simulink model "PubIfDecisionLSM_MDL"  (R2020b)
settings: configuration reference "DspaceConfig" (kept outside this file)
PostLoadFcn:
  | if any(exist('dsrtsu_mdlpostloadfcn', 'file') ~= 0), dsrtsu_mdlpostloadfcn('Execute', bdroot); end
InitFcn:
  | , if any(exist('rtifpga_mdlclblib', 'file') ~= 0), rtifpga_mdlclblib('Init', bdroot); end,
  | , if any(exist('dsmpb_private', 'file') ~= 0), dsmpb_private('dsmpb_mdlclblib', 'Init', bdroot); end,
values from neighbouring files (symbols this model uses):
  P_LSM_ALC_Enable = 0.0    [LSM_Parameter.sldd]
  P_LSM_AwayEdge_offset = 0.1    [LSM_Parameter.sldd]
  P_LSM_CentValidErr = 1.0    [LSM_Parameter.sldd]
  P_LSM_DOP_C0_EN_Limit = 0.8    [LSM_Parameter.sldd]
  P_LSM_DOP_C0_out_Limit = 2.0    [LSM_Parameter.sldd]
  P_LSM_DOP_C1_EN_Limit : value not decoded    [LSM_Parameter.sldd]
  P_LSM_DOP_C1_out_Limit : value not decoded    [LSM_Parameter.sldd]
  P_LSM_DOP_C1AndC2_Lim_X : value not decoded    [LSM_Parameter.sldd]
  P_LSM_DOP_C2_EN_Limit : value not decoded    [LSM_Parameter.sldd]
  P_LSM_DOP_C2_out_Limit : value not decoded    [LSM_Parameter.sldd]
  P_LSM_DOP_In_Pre2Dop_Dis = 1.0    [LSM_Parameter.sldd]
  P_LSM_DOP_Out_Pre2Dop_Dis = 2.0    [LSM_Parameter.sldd]
  P_LSM_DOP_PreDis_X : value not decoded    [LSM_Parameter.sldd]
  P_LSM_DOP_PreDis_Y : value not decoded    [LSM_Parameter.sldd]
  P_LSM_DOPEnableSW = 1.0    [LSM_Parameter.sldd]
  P_LSM_DOPValid_CheckTime = 0.06    [LSM_Parameter.sldd]
  P_LSM_DoubleLine_Curr2Cent_Dislimit = 0.5    [LSM_Parameter.sldd]
  P_LSM_DoubleLine_Dop2Cent_Dislimit = 0.5    [LSM_Parameter.sldd]
  P_LSM_DoubleLine_DOPOut_C1 : value not decoded    [LSM_Parameter.sldd]
  P_LSM_DoubleLine_Pre2Cent_Dislimit = 1.0    [LSM_Parameter.sldd]
  P_LSM_Error_Limit = 0.5    [LSM_Parameter.sldd]
  P_LSM_IFV2CenterAxis = 0.0    [LSM_Parameter.sldd]
  P_LSM_IFV2RearAxis = 0.0    [LSM_Parameter.sldd]
  P_LSM_Line2Edge_limit = 0.5    [LSM_Parameter.sldd]
  P_LSM_Line_Error = 0.1    [LSM_Parameter.sldd]
  P_LSM_LineSTD_Limit = 0.15    [LSM_Parameter.sldd]
  P_LSM_NOH_Switch = 0.0    [LSM_Parameter.sldd]
  P_LSM_OTL_C0_Factor = 1.0    [LSM_Parameter.sldd]
  P_LSM_OTL_C1_Factor = 0.5    [LSM_Parameter.sldd]
  P_LSM_OTL_C2_Factor = 0.5    [LSM_Parameter.sldd]
  P_LSM_Pre2OnlyLineDis = 5.0    [LSM_Parameter.sldd]
  P_LSM_Pre_t = 0.0    [LSM_Parameter.sldd]
  P_LSM_SingleLine_Cent2Edge_Dislimit = 100.0    [LSM_Parameter.sldd]
  P_LSM_SingleLine_Curr2Cent_Dislimit = 0.2    [LSM_Parameter.sldd]
  P_LSM_SingleLine_Dop2Cent_Dislimit = 0.2    [LSM_Parameter.sldd]
  P_LSM_SingleLine_DOPOut_C1 : value not decoded    [LSM_Parameter.sldd]
  P_LSM_SingleLine_Pre2Cent_Dislimit = 0.5    [LSM_Parameter.sldd]
  P_LSM_TJALimitSpd = 60.0    [LSM_Parameter.sldd]
undefined symbols (not defined in the file or in its folder): P_lCS_IFV2CenterAxis, P_LCS_IFV2RearAxis, P_LSM_EntryEdge_offset, P_LSM_EntryLnChngEnSwitch, P_LSM_EntryVanishDis, P_LSM_LinetLostTime, P_LSM_LineWijCal_C12, P_LSM_LineWijCal_C13, P_LSM_MapValid_ErrorSwitch, P_LSM_PosLineLcFac, P_LSM_SpdLim_Stub_Spd, P_LSM_SpdLim_StubLength, P_LSM_SpdTurnAlarm
libraries: simulink x324, TrueDurationTime x11
(part 8 of 25)

== system PubIfDecisionLSM_MDL/Subsystem1/TargetLineCalc_20ms/TargetLineCalc/DetectChange ==
  OTLCount : Inport
  Relational Operator : RelationalOperator  Operator=~=  OutDataTypeStr=boolean  RndMeth=Simplest
  Unit Delay49 : UnitDelay  InitialCondition=uint8(0)  SampleTime=-1  HasFrameUpgradeWarning=on
  Out1 : Outport
  wires:
  Unit Delay49/1 -> Relational Operator/1
  OTLCount/1 -> Relational Operator/2, Unit Delay49/1
  Relational Operator/1 -> Out1/1

== system PubIfDecisionLSM_MDL/Subsystem1/TargetLineCalc_20ms/TargetLineCalc/DetectIncrease ==
  LeftOffset_b : Inport
  Relational Operator : RelationalOperator  Operator=>  OutDataTypeStr=boolean  RndMeth=Simplest
  Unit Delay67 : UnitDelay  SampleTime=-1  HasFrameUpgradeWarning=on
  Out : Outport
  wires:
  Unit Delay67/1 -> Relational Operator/2
  LeftOffset_b/1 -> Unit Delay67/1, Relational Operator/1
  Relational Operator/1 -> Out/1

== system PubIfDecisionLSM_MDL/Subsystem1/TargetLineCalc_20ms/TargetLineCalc/DetectIncrease1 ==
  RightOffset_b : Inport
  Relational Operator : RelationalOperator  Operator=>  OutDataTypeStr=boolean  RndMeth=Simplest
  Unit Delay67 : UnitDelay  SampleTime=-1  HasFrameUpgradeWarning=on
  Out : Outport
  wires:
  Unit Delay67/1 -> Relational Operator/2
  RightOffset_b/1 -> Unit Delay67/1, Relational Operator/1
  Relational Operator/1 -> Out/1

== system PubIfDecisionLSM_MDL/Subsystem1/TargetLineCalc_20ms/TargetLineCalc/Subsystem2 ==
  LCKSts : Inport
  Line_State : Inport  Port=2
  vRef : Inport  Port=3
  DOP_Valid : Inport  Port=4
  DOP_C3 : Inport  Port=5
  DOP_C2 : Inport  Port=6
  DOP_C1 : Inport  Port=7
  DOP_C0 : Inport  Port=8
  DOP_Range : Inport  Port=9
  CentLine : Inport  Port=10
  EdgeLine : Inport  Port=11
  kap : Inport  Port=12
  Bus Selector1 : BusSelector  OutputSignals=EdgeConf,EdgeA3,EdgeA2,EdgeA1,EdgeA0
  Bus Selector6 : BusSelector  OutputSignals=PathValid,PathA3,PathA2,PathA1,PathA0,PathRange
  Constant11 : Constant  Value=1.3  OutDataTypeStr=single
  Constant13 : Constant  Value=P_LSM_DoubleLine_Dop2Cent_Dislimit
  Constant14 : Constant  Value=P_LSM_DOP_In_Pre2Dop_Dis
  Constant16 : Constant  Value=P_LSM_SingleLine_Cent2Edge_Dislimit
  Constant17 : Constant  Value=P_LSM_SingleLine_Pre2Cent_Dislimit
  Constant18 : Constant  Value=P_LSM_SingleLine_Curr2Cent_Dislimit
  Constant19 : Constant  Value=P_LSM_DoubleLine_Pre2Cent_Dislimit
  Constant20 : Constant  Value=P_LSM_DoubleLine_Curr2Cent_Dislimit
  Constant21 : Constant  Value=P_LSM_SingleLine_Dop2Cent_Dislimit
  Constant22 : Constant  Value=P_LSM_DOP_Out_Pre2Dop_Dis
  Constant23 : Constant  Value=P_LSM_DOPValid_CheckTime
  Constant3 : Constant  Value=P_LSM_DOP_C0_EN_Limit
  Constant6 : Constant  Value=P_LSM_DOP_C0_out_Limit
  Constant9 : Constant  Value=1.3  OutDataTypeStr=single
  Gain1 : Gain  Gain=3.6
  Gain2 : Gain  Gain=1.03
  Gain3 : Gain  Gain=3.6
  Gain4 : Gain  Gain=1.03
  LineSelect1 : MATLAB Function  TreatAsAtomicUnit=on
  MATLAB Function : MATLAB Function  TreatAsAtomicUnit=on
  Relational Operator3 : RelationalOperator  Operator=>  OutDataTypeStr=boolean  RndMeth=Simplest
  Selector{1..5,13} (6 alike) : Selector  InputPortWidth=3  IndexOptions=Index vector (dialog)  Indices=2  OutputSizes=1
  Sum : Sum  Inputs=|++
  Sum1 : Sum  Inputs=|++
  TJA_Line_Select : Stateflow chart  TreatAsAtomicUnit=on
      settings: PortSchema="{\"entries\":[{\"content\":{\"sides\":[{\"content\":{\"connectorIds\":[\"In4\",\"In5\",\"In1\",\"In3\",\"In6\",\"In2\"]},\"type\":\"ConnectorPlacement.EquallySpacedRectSide\",\"uuid\":\"94136a59-7eb8-456e-b1b6-1f0641166e38\"},{\"content\":{\"connectorIds\":[\"Out1\",\"Out2\"],\"side\":\"RIGHT\"},\"type\":\"ConnectorPlacement.EquallySpacedRectSide\",\"uuid\":\"664f3682-a903-47ba-a547-cb8bac6665aa\"},{\"content\":{\"connectorIds\":[],\"side\":\"TOP\"},\"type\":\"ConnectorPlacement.EquallySpacedRectSide\",\"uuid\":\"464c275d-d572-4c7f-987d-e7fbd4ad7b48\"},{\"content\":{\"connectorIds\":[],\"side\":\"HIDDEN\"},\"type\":\"ConnectorPlacement.EquallySpacedRectSide\",\"uuid\":\"4c0a197a-3630-40df-8db9-9313a36d3a51\"}]},\"type\":\"ConnectorPlacement.EquallySpacedConnector\",\"uuid\":\"5cfbbf76-c0d2-41e2-9bfb-a7f0229f0d71\"}],\"packageUris\":[\"http://schema.mathworks.com/mf0/Connector/R2020b\"],\"version\":\"1.0\"}"
  TrueDurationTime8 : TrueDurationTime/TrueDurationTime  TCycle=0.02
  Unit Delay : UnitDelay  SampleTime=-1  HasFrameUpgradeWarning=on
  Unit Delay1 : UnitDelay  SampleTime=-1  HasFrameUpgradeWarning=on
  Unit Delay2 : UnitDelay  SampleTime=-1  HasFrameUpgradeWarning=on
  preDisMinTable : Lookup_n-D  NumberOfTableDimensions=1  BreakpointsForDimension1=P_LSM_DOP_PreDis_X  Table=P_LSM_DOP_PreDis_Y  ExtrapMethod=Clip  InternalRulePriority=Speed  RndMeth=Simplest  InputSameDT=on
  preDisMinTable1 : Lookup_n-D  NumberOfTableDimensions=1  BreakpointsForDimension1=P_LSM_DOP_C1AndC2_Lim_X  Table=P_LSM_DOP_C1_EN_Limit  ExtrapMethod=Clip  InternalRulePriority=Speed  RndMeth=Simplest  InputSameDT=on
  preDisMinTable2 : Lookup_n-D  NumberOfTableDimensions=1  BreakpointsForDimension1=P_LSM_DOP_C1AndC2_Lim_X  Table=P_LSM_DOP_C2_EN_Limit  ExtrapMethod=Clip  InternalRulePriority=Speed  RndMeth=Simplest  InputSameDT=on
  preDisMinTable3 : Lookup_n-D  NumberOfTableDimensions=1  BreakpointsForDimension1=P_LSM_DOP_C1AndC2_Lim_X  Table=P_LSM_DOP_C1_out_Limit  ExtrapMethod=Clip  InternalRulePriority=Speed  RndMeth=Simplest  InputSameDT=on
  preDisMinTable4 : Lookup_n-D  NumberOfTableDimensions=1  BreakpointsForDimension1=P_LSM_DOP_C1AndC2_Lim_X  Table=P_LSM_DOP_C2_out_Limit  ExtrapMethod=Clip  InternalRulePriority=Speed  RndMeth=Simplest  InputSameDT=on
  preDisMinTable5 : Lookup_n-D  NumberOfTableDimensions=1  BreakpointsForDimension1=P_LSM_DOP_C1AndC2_Lim_X  Table=P_LSM_DoubleLine_DOPOut_C1  ExtrapMethod=Clip  InternalRulePriority=Speed  RndMeth=Simplest  InputSameDT=on
  preDisMinTable7 : Lookup_n-D  NumberOfTableDimensions=1  BreakpointsForDimension1=P_LSM_DOP_C1AndC2_Lim_X  Table=P_LSM_SingleLine_DOPOut_C1  ExtrapMethod=Clip  InternalRulePriority=Speed  RndMeth=Simplest  InputSameDT=on
  vRef2 : InportShadow  Port=3
  OTL_Valid : Outport
  OTL_C3 : Outport  Port=2
  OTL_C2 : Outport  Port=3
  OTL_C1 : Outport  Port=4
  OTL_C0 : Outport  Port=5
  OTL_Range : Outport  Port=6
  TJA_Line_State : Outport  Port=7
  Line_source : Outport  Port=8
  wires:
  [SpeedKph] -> preDisMinTable7/1, preDisMinTable5/1
  preDisMinTable7/1 -> LineSelect1/27(SingleLine_DOPOut_C1)
  preDisMinTable5/1 -> LineSelect1/28(DoubleLine_DOPOut_C1)
  preDisMinTable2/1 -> MATLAB Function/7(DOP_C2_EN_Limit)
  preDisMinTable1/1 -> MATLAB Function/6(DOP_C1_EN_Limit)
  preDisMinTable3/1 -> MATLAB Function/9(DOP_C1_out_Limit)
  [SpeedKph] -> preDisMinTable1/1, preDisMinTable2/1, preDisMinTable3/1, preDisMinTable4/1
  Unit Delay2/1 -> MATLAB Function/14(dy_pre)
  LineSelect1/7(dy_pre) -> Unit Delay2/1
  Unit Delay1/1 -> MATLAB Function/15(Y_DOP)
  LineSelect1/5(Cent2DOP_flag) -> TJA_Line_Select/6(Cent2DOP_flag)
  LineSelect1/6(DOP2Cent_flag) -> TJA_Line_Select/2(DOP2Cent_flag)
  Unit Delay/1 -> MATLAB Function/1(TJA_Line)
  MATLAB Function/2(DOP_Out_Enable) -> LineSelect1/31(DOP_OUT)  "LSM_DOP_Out"
  Constant23/1 -> Relational Operator3/2
  Constant22/1 -> MATLAB Function/12(DOP_Out_Pre2Dop_Dis)
  Constant21/1 -> LineSelect1/26(SingleLine_Dop2Cent_Dislimit)
  Constant18/1 -> LineSelect1/25(SingleLine_Curr2Cent_Dislimit)
  Constant17/1 -> LineSelect1/24(SingleLine_Pre2Cent_Dislimit)
  Constant16/1 -> LineSelect1/23(SingleLine_Cent2Edge_Dislimit)
  LineSelect1/4(DOP2Off_flag) -> TJA_Line_Select/3(DOP2Off_flag)
  LineSelect1/3(Cent2Off_flag) -> TJA_Line_Select/1(Cent2Off_flag)
  LineSelect1/2(Off2DOP_flag) -> TJA_Line_Select/5(Off2DOP_flag)
  LineSelect1/1(Off2Cent_flag) -> TJA_Line_Select/4(Off2Cent_flag)
  kap/1 -> LineSelect1/3(kap)
  Constant13/1 -> LineSelect1/22(DoubleLine_Dop2Cent_Dislimit)
  Constant20/1 -> LineSelect1/21(DoubleLine_Curr2Cent_Dislimit)
  Constant19/1 -> LineSelect1/20(DoubleLine_Pre2Cent_Dislimit)
  EdgeLine/1 -> Bus Selector1/1
  Bus Selector1/1 -> LineSelect1/15(VisEdgeConf)  "<EdgeConf>"
  Bus Selector1/3 -> LineSelect1/17(VisEdgeA2)  "<EdgeA2>"
  Bus Selector1/5 -> LineSelect1/19(VisEdgeA0)  "<EdgeA0>"
  Bus Selector1/2 -> LineSelect1/16(VisEdgeA3)  "<EdgeA3>"
  Bus Selector1/4 -> LineSelect1/18(VisEdgeA1)  "<EdgeA1>"
  [DOP_C2] -> LineSelect1/12(bOTL)
  [DOP_C1] -> LineSelect1/13(cOTL)
  [DOP_C0] -> LineSelect1/14(dOTL)
  [DOP_C3] -> LineSelect1/11(aOTL)
  Bus Selector6/3 -> Selector2/1  "<PathA2>"
  Bus Selector6/6 -> Selector5/1  "<PathRange>"
  Bus Selector6/5 -> Selector4/1  "<PathA0>"
  Bus Selector6/1 -> Selector13/1  "<PathValid>"
  Bus Selector6/2 -> Selector1/1  "<PathA3>"
  Bus Selector6/4 -> Selector3/1  "<PathA1>"
  CentLine/1 -> Bus Selector6/1
  Constant14/1 -> MATLAB Function/11(DOP_In_Pre2Dop_Dis)
  LineSelect1/8(Y_DOP) -> Unit Delay1/1
  Line_State/1 -> LineSelect1/2(Line_State)
  Gain1/1 -> Gain2/1
  Sum1/1 -> preDisMinTable/1
  vRef2/1 -> Gain1/1
  Gain2/1 -> Sum1/1
  Constant11/1 -> Sum1/2
  LCKSts/1 -> LineSelect1/4(LCKSts)
  preDisMinTable/1 -> LineSelect1/1(Pre_dis)
  Constant9/1 -> Sum/2
  vRef/1 -> Gain3/1
  Gain4/1 -> Sum/1
  Gain3/1 -> Gain4/1
  Sum/1 -> LineSelect1/29(Vehicle_Speed), [SpeedKph]
  Relational Operator3/1 -> MATLAB Function/13(DOP_Valid)
  TrueDurationTime8/1 -> Relational Operator3/1
  [DOP_Valid] -> TrueDurationTime8/1
  preDisMinTable4/1 -> MATLAB Function/10(DOP_C2_out_Limit)
  Constant6/1 -> MATLAB Function/8(DOP_CO_out_Limit)
  Constant3/1 -> MATLAB Function/5(DOP_CO_EN_Limit)
  TJA_Line_Select/1(TJA_Line) -> TJA_Line_State/1, Unit Delay/1
  MATLAB Function/1(DOP_In_Enable) -> LineSelect1/30(DOP_EN)  "LSM_DOP_EN"
  DOP_C0/1 -> OTL_C0/1, [DOP_C0]
  DOP_Valid/1 -> [DOP_Valid], OTL_Valid/1
  DOP_Range/1 -> OTL_Range/1, [DOP_Range]
  DOP_C1/1 -> OTL_C1/1, [DOP_C1]
  DOP_C2/1 -> OTL_C2/1, [DOP_C2]
  DOP_C3/1 -> OTL_C3/1, [DOP_C3]
  [DOP_C0] -> MATLAB Function/2(DOP_CO)
  [DOP_C1] -> MATLAB Function/3(DOP_C1)
  [DOP_C2] -> MATLAB Function/4(DOP_C2)
  Selector13/1 -> LineSelect1/5(CentLaneValid)
  Selector1/1 -> LineSelect1/6(CentLineA3)
  Selector2/1 -> LineSelect1/7(CentLineA2)
  Selector3/1 -> LineSelect1/8(CentLineA1)
  Selector4/1 -> LineSelect1/9(CentLineA0)
  Selector5/1 -> LineSelect1/10(CentRange)
  TJA_Line_Select/2(TJA_Source) -> Line_source/1

== system PubIfDecisionLSM_MDL/Subsystem1/TargetLineCalc_20ms/TargetLineCalc/Subsystem3 ==
  Intersec_available : Inport
  f_distance : Inport  Port=2  OutDataTypeStr=single
  en_direction : Inport  Port=3  OutDataTypeStr=uint8
  i_rec_lanes_num : Inport  Port=4  OutDataTypeStr=uint8
  i_rec_lanes : Inport  Port=5  OutDataTypeStr=uint8
  nLaneNum : Inport  Port=6  OutDataTypeStr=uint8
  nLaneID : Inport  Port=7  OutDataTypeStr=uint8
  i_mapvalid : Inport  Port=8  OutDataTypeStr=uint8
  i_on_nav_path : Inport  Port=9  OutDataTypeStr=uint8
  " b_vanish_valid" : Inport  Port=10  OutDataTypeStr=boolean
  " Exit_dDisStart" : Inport  Port=11  OutDataTypeStr=single
  ExitLineExist : Inport  Port=12  OutDataTypeStr=uint8
  " Exit_dC0V" : Inport  Port=13  OutDataTypeStr=single
  RoadType : Inport  Port=14  OutDataTypeStr=uint8
  VehInLeftmostLane : Inport  Port=15  OutDataTypeStr=boolean
  VehInRightmostLane : Inport  Port=16  OutDataTypeStr=boolean
  Entry_bIsLineExist : Inport  Port=17
  Entry_dDisStart : Inport  Port=18
  Entry_dC0V : Inport  Port=19
  " f_vanish_pt_dis " : Inport  Port=20
  Subsystem : Subsystem
  Subsystem2 : Subsystem
  Subsystem3 : Subsystem
  PilotRoadSts : Outport  OutDataTypeStr=uint8
  PilotTurnSwSts : Outport  Port=2  OutDataTypeStr=uint8
  PilotSts : Outport  Port=3  OutDataTypeStr=uint8
  LaneChange : Outport  Port=4  OutDataTypeStr=uint8
  LSM_PilotSPL : Outport  Port=5  OutDataTypeStr=uint8
  PilotSPLDist : Outport  Port=6  OutDataTypeStr=uint16
  wires:
  " b_vanish_valid"/1 -> Subsystem2/11(" b_vanish_valid")
  nLaneNum/1 -> Subsystem2/9(nLaneNum)
  VehInLeftmostLane/1 -> Subsystem2/8(VehInLeftmostLane)
  VehInRightmostLane/1 -> Subsystem2/7(VehInRightmostLane)
  RoadType/1 -> Subsystem/3(RoadType)
  nLaneID/1 -> Subsystem2/5(nLaneID), [nLaneID]
  i_on_nav_path/1 -> Subsystem/2(i_on_nav_path)
  " Exit_dC0V"/1 -> Subsystem2/13(Exit_dC0V)
  " Exit_dDisStart"/1 -> Subsystem2/12(" Exit_dDisStart")
  f_distance/1 -> Subsystem2/2(f_distance), Subsystem/5(f_distance)
  Subsystem2/9(rExitStub3) -> Subsystem/14(rExitStub3)
  i_rec_lanes_num/1 -> Subsystem2/10(i_rec_lanes_num)
  i_mapvalid/1 -> Subsystem/1(i_mapvalid)
  i_rec_lanes/1 -> Subsystem2/4(i_rec_lanes)
  ExitLineExist/1 -> Subsystem2/1(Exit_bIsLineExist), Subsystem/4(bIsLineExist)
  en_direction/1 -> Subsystem2/6(en_direction)
  Subsystem2/16(lExitStub3) -> Subsystem/21(lExitStub3)
  Intersec_available/1 -> Subsystem2/3(b_is_available)
  Entry_bIsLineExist/1 -> Subsystem2/14(Entry_bIsLineExist)
  Entry_dDisStart/1 -> Subsystem2/15(Entry_dDisStart)
  Entry_dC0V/1 -> Subsystem2/16(Entry_dC0V)
  Subsystem/2(PilotTurnSwSts) -> [PilotTurnSwSts], PilotTurnSwSts/1
  Subsystem2/1(StubValid) -> Subsystem/6(StubValid)
  Subsystem2/2(RightStub) -> Subsystem/7(RightStub)
  Subsystem2/3(LeftStub) -> Subsystem/8(LeftStub)
  Subsystem2/4(CruiseValid) -> Subsystem/9(CruiseValid)
  Subsystem2/5(TurnLeft) -> Subsystem/10(TurnLeft)
  Subsystem2/6(TurnRight) -> Subsystem/11(TurnRight)
  Subsystem2/7(rExitStub1) -> Subsystem/12(rExitStub1)
  Subsystem2/8(rExitStub2) -> Subsystem/13(rExitStub2)
  Subsystem2/10(Vanish_turnleft) -> Subsystem/15(Vanish_turnleft)
  Subsystem2/11(EntryStub1) -> Subsystem/16(EntryStub1)
  Subsystem2/12(CruiseRight) -> Subsystem/17(CruiseRight)
  Subsystem2/13(CruiseLeft) -> Subsystem/18(CruiseLeft)
  Subsystem2/14(lExitStub1) -> Subsystem/19(lExitStub1)
  Subsystem2/15(lExitStub2) -> Subsystem/20(lExitStub2)
  Subsystem2/17(CruiseTurn) -> Subsystem/22(CruiseTurn)
  Subsystem2/18(Forbid_TurnRight) -> Subsystem/23(FrbRight)
  Subsystem2/19(Forbid_TurnLeft) -> Subsystem/24(FrbLeft)
  Subsystem2/20(OneLane) -> Subsystem/25(OneLane)
  Subsystem2/21(EntryStub2) -> Subsystem/26(EntryStub2)
  Subsystem2/22(EntryStub3) -> Subsystem/27(EntryStub3)
  Subsystem2/23(EntryStub4) -> Subsystem/28(EntryStub4)
  Subsystem2/24(EntryStub5) -> Subsystem/29(EntryStub5)
  Subsystem2/25(EntryStub6) -> Subsystem/30(EntryStub6)
  Subsystem2/26(EntryStub5_TurnLeft) -> Subsystem/31(EntryStub5_TurnLeft)
  Subsystem/1(PilotRoadSts) -> PilotRoadSts/1
  Subsystem/3(LSM_PilotSPL) -> LSM_PilotSPL/1
  Subsystem/4(PilotSPLDist) -> PilotSPLDist/1
  " f_vanish_pt_dis "/1 -> Subsystem2/17(" f_vanish_pt_dis ")
  Subsystem3/1(LaneChange) -> LaneChange/1
  Subsystem2/27(rExitStub4_takeover) -> Subsystem/32(rExitStub4_takeover)
  Subsystem2/28(lExitStub4_takeover) -> Subsystem/33(lExitStub4_takeover)
  Subsystem2/29(EntryStub5_takeover) -> Subsystem/34(EntryStub5_takeover)
  Subsystem2/30(Vanish_turnleft_takeover) -> Subsystem/35(Vanish_turnleft_takeover)
  Subsystem/5(PilotSts) -> PilotSts/1
  [PilotTurnSwSts] -> Subsystem3/1(PilotTurnSwSts)
  [nLaneID] -> Subsystem3/2(nLaneID)

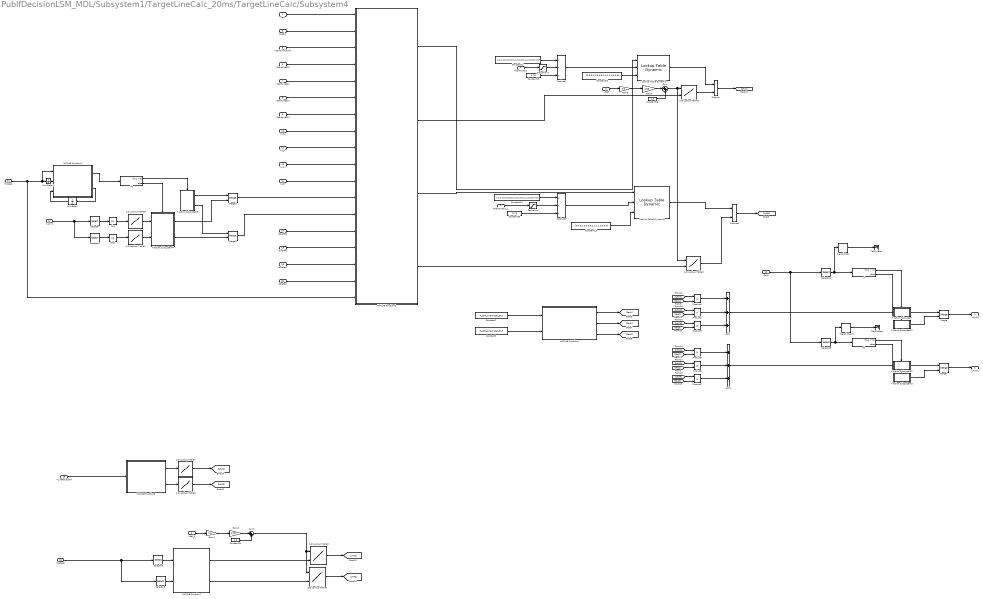
== system PubIfDecisionLSM_MDL/Subsystem1/TargetLineCalc_20ms/TargetLineCalc/Subsystem4 ==
  kap : Inport
  vRef : Inport  Port=2
  preDis : Inport  Port=3
  RoadWidth1 : Inport  Port=4
  <CentLineValid> : Inport  Port=5
  <CentLineC3> : Inport  Port=6
  <CentLineC2> : Inport  Port=7
  <CentLineC1> : Inport  Port=8
  <CentLineC0> : Inport  Port=9
  Conf : Inport  Port=10
  <A3> : Inport  Port=11
  <A2> : Inport  Port=12
  <A1> : Inport  Port=13
  <A0> : Inport  Port=14
  <LineReliable> : Inport  Port=15
  <Range> : Inport  Port=16
  CosOfPsi : Inport  Port=17
  SinOfPsi : Inport  Port=18
  dDeltaX : Inport  Port=19
  dDeltaY : Inport  Port=20
  HWASts : Inport  Port=21
  1-D Lookup Table1 : Lookup_n-D  NumberOfTableDimensions=1  BreakpointsForDimension1=[0 0.0001 0.0005 0.001 0.005 0.01 0.05]  Table=[0 0.1 0.3 0.6 0.8 0.8 0.8]  InternalRulePriority=Speed  RndMeth=Simplest  InputSameDT=on
  1-D Lookup Table3 : Lookup_n-D  NumberOfTableDimensions=1  BreakpointsForDimension1=[0 0.0001 0.0005 0.001 0.005 0.01 0.05]  Table=[0 0.1 0.3 0.6 0.8 0.8 0.8]  InternalRulePriority=Speed  RndMeth=Simplest  InputSameDT=on
  1-D Lookup Table5 : Lookup_n-D  NumberOfTableDimensions=1  BreakpointsForDimension1=[0 0.1 0.3 0.5 0.7 0.9 1]  Table=[0 0.1 0.2 0.4 0.7 1 1]  InternalRulePriority=Speed  RndMeth=Simplest  InputSameDT=on
  1-D Lookup Table6 : Lookup_n-D  NumberOfTableDimensions=1  BreakpointsForDimension1=[0 0.1 0.3 0.5 0.7 0.9 1]  Table=[0 0.1 0.2 0.4 0.7 1 1]  InternalRulePriority=Speed  RndMeth=Simplest  InputSameDT=on
  2-D Lookup Table2 : Lookup_n-D  BreakpointsForDimension1=[20,50,100,120]  BreakpointsForDimension2=[0,0.2,0.4,0.6,0.8,1,1.2,1.4,1.6,1.8,2,2.5,3]  Table=reshape([1,1,1,1,1,1,1,1,1,1,1,1,1,1,1,0.8,1,0.9,0.5,0.4,1,0.8,0.3,0.2,1,0.7,0.1,0.1,1,0.6,0,0,0.8,0.5,0,0,0.7,0.3,0,0,0.6,0,0,0,0.3,0,0,0,0,0,0,0],4,13)  InternalRulePriority=Speed  RndMeth=Simplest  InputSameDT=on
      settings: InputPortMap=u0,u1
  2-D Lookup Table3 : Lookup_n-D  BreakpointsForDimension1=[10,50,80,120]  BreakpointsForDimension2=[0,5,10,20,40,50,60,80,100]  Table=reshape([0,0,0,0,0,0,0,0,0.4,0.2,0,0,0.6,0.4,0.2,0,1,0.6,0.5,0.3,1,0.8,0.7,0.5,1,1,0.9,0.8,1,1,1,1,1,1,1,1],4,9)  InternalRulePriority=Speed  RndMeth=Simplest  InputSameDT=on
      settings: InputPortMap=u0,u1
  2-D Lookup Table4 : Lookup_n-D  BreakpointsForDimension1=[10,50,80,120]  BreakpointsForDimension2=[0,5,10,20,40,50,60,80,100]  Table=reshape([0,0,0,0,0,0,0,0,0.4,0.2,0,0,0.6,0.4,0.2,0,1,0.6,0.5,0.3,1,0.8,0.7,0.5,1,1,0.9,0.8,1,1,1,1,1,1,1,1],4,9)  InternalRulePriority=Speed  RndMeth=Simplest  InputSameDT=on
      settings: InputPortMap=u0,u1
  2-D Lookup Table5 : Lookup_n-D  BreakpointsForDimension1=[20,50,100,120]  BreakpointsForDimension2=[0,0.2,0.4,0.6,0.8,1,1.2,1.4,1.6,1.8,2,2.5,3]  Table=reshape([1,1,1,1,1,1,1,1,1,1,1,1,1,1,1,0.8,1,0.9,0.5,0.4,1,0.8,0.3,0.2,1,0.7,0.1,0.1,1,0.6,0,0,0.8,0.5,0,0,0.7,0.3,0,0,0.6,0,0,0,0.3,0,0,0,0,0,0,0],4,13)  InternalRulePriority=Speed  RndMeth=Simplest  InputSameDT=on
      settings: InputPortMap=u0,u1
  <A2>1 : InportShadow  Port=12
  Abs : Abs
  Abs1 : Abs
  Add : Sum  Inputs=+++
  Add1 : Sum  Inputs=+++
  Constant10 : Constant  Value=[0,0,0.2,0.5,0.8,1,1,1,1,0.3,0,0]
  Constant11 : Constant  Value=[-1.2,-0.2,0,0.5,1,1.3,1.5,2.1,2.3,3.5,4,5]
  Constant12 : Constant  Value=3.75
  Constant13 : Constant  Value=[0,0,0.2,0.5,0.8,1,1,1,1,0.3,0,0]
  Constant14 : Constant  Value=[-1.2,-0.2,0,0.5,1,1.3,1.5,2.1,2.3,3.5,4,5]
  Constant15 : Constant  Value=3.75
  Constant16 : Constant  Value=1.3  OutDataTypeStr=single
  Constant21 : Constant  Value=1.3  OutDataTypeStr=single
  Constant7 : Constant  Value=P_LSM_LineWijCal_C12
  Constant9 : Constant  Value=P_LSM_LineWijCal_C13
  Gain1 : Gain  Gain=3.6
  Gain2 : Gain  Gain=1.03
  Gain3 : Gain  Gain=3.6
  Gain4 : Gain  Gain=1.03
  If : If
  If Action Subsystem : Subsystem  TreatAsAtomicUnit=on
  If Action Subsystem1 : Subsystem  TreatAsAtomicUnit=on
  If Action Subsystem2 : Subsystem  TreatAsAtomicUnit=on
  If Action Subsystem3 : Subsystem  TreatAsAtomicUnit=on
  If Action Subsystem4 : Subsystem  TreatAsAtomicUnit=on
  If Action Subsystem5 : Subsystem  TreatAsAtomicUnit=on
  If1 : If
  If2 : If
  Lookup Table Dynamic : simulink/Lookup Tables/Lookup Table Dynamic  LookUpMeth=Interpolation-Use End Values  OutDataType=fixdt('single')  OutScaling=[]  OutputDataTypeScalingMode=Specify via dialog  OutDataTypeStr=single  DoSatur=off
  Lookup Table Dynamic1 : simulink/Lookup Tables/Lookup Table Dynamic  LookUpMeth=Interpolation-Use End Values  OutDataType=fixdt('single')  OutScaling=[]  OutputDataTypeScalingMode=Specify via dialog  OutDataTypeStr=single  DoSatur=off
  MATLAB Function2 : MATLAB Function  TreatAsAtomicUnit=on
  MATLAB Function3 : MATLAB Function  TreatAsAtomicUnit=on
  MATLAB Function6 : MATLAB Function  TreatAsAtomicUnit=on
  MATLAB Function7 : MATLAB Function  TreatAsAtomicUnit=on
  MATLAB Function8 : MATLAB Function  TreatAsAtomicUnit=on
  Merge{,1..3} (4 alike) : Merge
  Product{,1..7} (8 alike) : Product
  Product8 : Product  Inputs=**/
  Product9 : Product  Inputs=**/
  RoadWidth1_1 : InportShadow  Port=4
  Saturation : Saturate  UpperLimit=single(5)  LowerLimit=single(2.4)
  Saturation1 : Saturate  UpperLimit=single(5)  LowerLimit=single(2.4)
  Selector : Selector  InputPortWidth=4  IndexOptions=Index vector (dialog)  Indices=2  OutputSizes=1
  Selector1 : Selector  InputPortWidth=4  IndexOptions=Index vector (dialog)  Indices=3  OutputSizes=1
  Selector2 : Selector  InputPortWidth=4  IndexOptions=Index vector (dialog)  Indices=2  OutputSizes=1
  Selector3 : Selector  InputPortWidth=4  IndexOptions=Index vector (dialog)  Indices=3  OutputSizes=1
  Selector4 : Selector  InputPortWidth=4  IndexOptions=Index vector (dialog)  Indices=2  OutputSizes=1
  Selector5 : Selector  InputPortWidth=4  IndexOptions=Index vector (dialog)  Indices=3  OutputSizes=1
  Signal Copy : SignalConversion  OverrideOpt=off
  Signal Copy1 : SignalConversion  OverrideOpt=off
  Sum : Sum  Inputs=|++
  Sum1 : Sum  Inputs=|++
  Terminator : Terminator
  Terminator1 : Terminator
  Unit Delay : UnitDelay  SampleTime=-1  HasFrameUpgradeWarning=on
  Unit Delay1 : UnitDelay  SampleTime=-1  HasFrameUpgradeWarning=on
  vRef_1 : InportShadow  Port=2
  LH1Wij : Outport
  LH2Wij : Outport  Port=2
  wires:
  Saturation1/1 -> Product8/2
  Saturation/1 -> Product9/2
  <CentLineValid>/1 -> MATLAB Function6/3(CentLineValidK1)
  If1/1 -> If Action Subsystem1/Action
  If/1 -> If Action Subsystem/Action
  If1/2 -> If Action Subsystem3/Action
  Add1/1 -> If Action Subsystem1/1(In1)
  Merge1/1 -> LH2Wij/1
  If Action Subsystem1/1(LH1Wij) -> Merge1/1
  If Action Subsystem3/1(LH1Wij) -> Merge1/2
  If Action Subsystem2/1(LH1Wij) -> Merge/2
  If Action Subsystem/1(LH1Wij) -> Merge/1
  Merge/1 -> LH1Wij/1
  If/2 -> If Action Subsystem2/Action
  Add/1 -> If Action Subsystem/1(In1)
  Selector4/1 -> Signal Copy/1, If/1
  Selector5/1 -> Signal Copy1/1, If1/1
  Conf/1 -> Selector4/1, Selector5/1
  dDeltaY/1 -> MATLAB Function6/17(dDeltaY)
  <A3>/1 -> MATLAB Function6/8(VisLineA3)
  <A1>/1 -> MATLAB Function6/10(VisLineA1)
  CosOfPsi/1 -> MATLAB Function6/14(CosOfPsi)
  Selector3/1 -> MATLAB Function7/2(L3_R)
  <A2>/1 -> MATLAB Function6/9(VisLineA2)
  Product3/1 -> Add/3
  MATLAB Function7/2(dy3_Ran) -> 2-D Lookup Table4/2
  2-D Lookup Table4/1 -> [LH32]  "LSM_LH32"
  kap/1 -> MATLAB Function6/1(kap)
  MATLAB Function3/3(Fac3) -> [Fac3]
  vRef/1 -> Gain3/1
  Product4/1 -> [LH31]  "LSM_LH31"
  MATLAB Function3/2(Fac2) -> [Fac2]
  preDis/1 -> MATLAB Function6/2(preDis)
  MATLAB Function8/1(dy2_Rel) -> 1-D Lookup Table5/1
  MATLAB Function7/1(dy2_Ran) -> 2-D Lookup Table3/2
  Constant15/1 -> Product9/3
  Constant7/1 -> MATLAB Function3/1(C12)
  [Fac3] -> Product3/2
  Abs/1 -> 1-D Lookup Table3/1
  [LH31] -> Product5/1
  Constant9/1 -> MATLAB Function3/2(C13)
  [Fac2] -> Product2/2
  MATLAB Function6/4(delta_d3) -> 2-D Lookup Table5/2  "LSM_DeltaDis3"
  [LH32] -> Product6/1
  <CentLineC3>/1 -> MATLAB Function6/4(CentLineC3K1)
  Constant10/1 -> Lookup Table Dynamic/3
  Lookup Table Dynamic/1 -> Product/1
  Constant14/1 -> Product9/1
  RoadWidth1_1/1 -> Saturation/1
  MATLAB Function6/2(delta_d2) -> 2-D Lookup Table2/2  "LSM_DeltaDis2"
  MATLAB Function6/3(d_cur3) -> Lookup Table Dynamic1/1  "LSM_CurDis3"
  Gain4/1 -> Sum/1
  Product6/1 -> Add1/2
  Constant11/1 -> Product8/1
  <A0>/1 -> MATLAB Function6/11(VisLineA0)
  Gain3/1 -> Gain4/1
  Product9/1 -> Lookup Table Dynamic1/2
  Selector2/1 -> MATLAB Function7/1(L2_R)
  <CentLineC1>/1 -> MATLAB Function6/6(CentLineC1K1)
  2-D Lookup Table2/1 -> Product/2
  Product1/1 -> Add/1
  [Fac1] -> Product1/2
  Product2/1 -> Add/2
  1-D Lookup Table6/1 -> [LH33]  "LSM_LH33"
  Product8/1 -> Lookup Table Dynamic/2
  SinOfPsi/1 -> MATLAB Function6/15(SinOfPsi)
  Selector1/1 -> Abs1/1
  [LH23] -> Product3/1
  <CentLineC2>/1 -> MATLAB Function6/5(CentLineC2K1)
  [Fac2] -> Product6/2
  [Fac1] -> Product5/2
  [Fac3] -> Product7/2
  Constant12/1 -> Product8/3
  Sum/1 -> 2-D Lookup Table5/1, 2-D Lookup Table2/1
  2-D Lookup Table3/1 -> [LH22]  "LSM_LH22"
  MATLAB Function3/1(Fac1) -> [Fac1]
  Constant21/1 -> Sum1/2
  Selector/1 -> Abs/1
  Constant13/1 -> Lookup Table Dynamic1/3
  Constant16/1 -> Sum/2
  MATLAB Function8/2(dy3_Rel) -> 1-D Lookup Table6/1
  dDeltaX/1 -> MATLAB Function6/16(dDeltaX)
  [LH33] -> Product7/1
  Product7/1 -> Add1/3
  1-D Lookup Table5/1 -> [LH23]  "LSM_LH23"
  Product5/1 -> Add1/1
  Sum1/1 -> 2-D Lookup Table3/1, 2-D Lookup Table4/1
  <LineReliable>/1 -> MATLAB Function8/1(VisLineReliable)
  2-D Lookup Table5/1 -> Product4/2
  MATLAB Function6/1(d_cur2) -> Lookup Table Dynamic/1  "LSM_CurDis2"
  vRef_1/1 -> Gain1/1
  RoadWidth1/1 -> Saturation1/1
  <Range>/1 -> Selector2/1, Selector3/1
  Product/1 -> [LH21]  "LSM_LH21"
  Gain2/1 -> Sum1/1
  <CentLineC0>/1 -> MATLAB Function6/7(CentLineC0K1)
  [LH21] -> Product1/1
  Gain1/1 -> Gain2/1
  Abs1/1 -> 1-D Lookup Table1/1
  Lookup Table Dynamic1/1 -> Product4/1
  [LH22] -> Product2/1
  MATLAB Function2/1(Changelane) -> If2/1
  If2/1 -> If Action Subsystem5/Action
  <A2>1/1 -> Selector1/1, Selector/1
  1-D Lookup Table3/1 -> If Action Subsystem4/1(In1)
  1-D Lookup Table1/1 -> If Action Subsystem4/2(In2)
  If2/2 -> If Action Subsystem4/Action
  If Action Subsystem5/1(Out1) -> Merge2/1
  If Action Subsystem4/2(Out2) -> Merge3/2
  If Action Subsystem4/1(Out1) -> Merge2/2
  If Action Subsystem5/2(Out2) -> Merge3/1
  Merge2/1 -> MATLAB Function6/12(n1)
  Merge3/1 -> MATLAB Function6/13(n2)
  Unit Delay1/1 -> MATLAB Function2/2(HWAStsK1)
  MATLAB Function2/2(Lock_counter) -> Unit Delay/1
  Unit Delay/1 -> MATLAB Function2/3(Lock_counterK1)
  HWASts/1 -> MATLAB Function6/18(HWASts), MATLAB Function2/1(HWASts), Unit Delay1/1
  Signal Copy/1 -> Terminator/1  "LSM_LeftLineConf"
  Signal Copy1/1 -> Terminator1/1  "LSM_RightLineConf"
